simulink model "Filter_FIR"  (Simulink 9.1)
settings: Solver=VariableStepAuto  StartTime=0.0  StopTime=1  RelTol=1e-3
values from neighbouring files (symbols this model uses):
  G = 10^(2/20)    (= 1.25892541179)    [FIR_Filtering.m]
libraries: dspfdesign x1
settings Model: Creator=Daniel  LastModifiedBy=Daniel
settings DataIOCC: SaveFormat=Dataset
settings OptimizationCC: LifeSpan=auto
settings DebuggingCC: UnderspecifiedInitializationDetection=Simplified  MergeDetectMultiDrivingBlocksExec=error  SFUnexpectedBacktrackingDiag=error  SFNoUnconditionalDefaultTransitionDiag=error  SFExecutionAtInitializationDiag=warning
settings HardwareCC: ProdBitPerPointer=64  ProdBitPerSizeT=64  ProdBitPerPtrDiffT=64  ProdLargestAtomicFloat=Float  ProdIntDivRoundTo=Zero  ProdEndianess=LittleEndian  ProdWordSize=64  ProdHWDeviceType=Intel->x86-64 (Windows64)
settings ModelReferenceCC: PropagateSignalLabelsOutOfModel=on
settings CodeAppCC: StateflowObjectComments=off
settings GRTTargetCC: TargetLangStandard=C99 (ISO)  CombineOutputUpdateFcns=on  GRTInterface=off
settings ConfigComp: CovMetricSettings=dwe  CovHtmlReporting=off  CovSaveCumulativeToWorkspaceVar=off  CovSaveSingleToWorkspaceVar=off  CovExternalEMLEnable=on

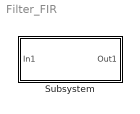
== system Filter_FIR ==
  Subsystem : Subsystem

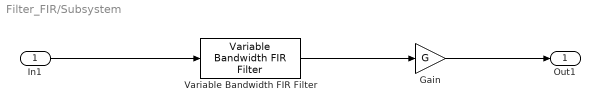
== system Filter_FIR/Subsystem ==
  In1 : Inport  OutDataTypeStr=double
  Gain : Gain  Gain=G
  Variable Bandwidth FIR Filter : dspfdesign/Variable Bandwidth FIR Filter  FilterOrder=30  FilterType=Bandpass  CutoffFrequencyPort=off  CutoffFrequency=512  CenterFrequencyPort=off  CenterFrequency=3500  BandwidthPort=off  Bandwidth=1000  Window=Hamming  KaiserWindowParameter=.5  SidelobeAttenuation=60  InheritSampleRate=off  SampleRate=Fs  SimulateUsing=Code generation
      settings: SourceProductName=DSP System Toolbox  SourceProductBaseCode=DS
  Out1 : Outport
  wires:
  In1/1 -> Variable Bandwidth FIR Filter/1
  Gain/1 -> Out1/1
  Variable Bandwidth FIR Filter/1 -> Gain/1
